simulink model "jointSpaceTrajController_reachPos"  (Simulink 8.0)
settings: Solver=FixedStepDiscrete  StartTime=0.0  StopTime=inf  FixedStep=Ts  RelTol=1e-3
undefined symbols (not defined in the file or in its folder): dqErr, qErr, qInit, qjDes, refMask, ROBOT_DOF
libraries: WBCLibrary x5
settings Model: Creator=nunoguedelha  LastModifiedBy=nunoguedelha

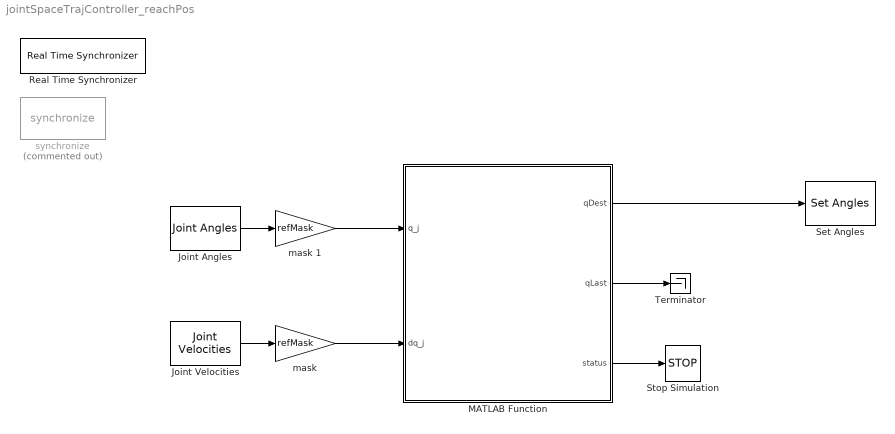
== system jointSpaceTrajController_reachPos ==
  Joint Angles : WBCLibrary/wholeBodyStates/Joint Angles  robotName=robotName  localName=localName
  Joint Velocities : WBCLibrary/wholeBodyStates/Joint Velocities  robotName=robotName  localName=localName
  MATLAB Function : MATLAB Function  TreatAsAtomicUnit=on
  Real Time Synchronizer : WBCLibrary/Utilities/Real Time Synchronizer  Priority=-10  threadPeriod=Ts
  Set Angles : WBCLibrary/wholeBodyActuators/Set Angles  val=5  robotName=robotName  localName=localName
  Stop Simulation : Stop
  Terminator : Terminator
  mask : Gain  Gain=refMask
  mask 1 : Gain  Gain=refMask
  synchronize : WBCLibrary/Utilities/synchronize  Commented=on  rate=0.010  scaleFactor=1
  wires:
  Joint Angles/1 -> mask 1/1
  Joint Velocities/1 -> mask/1
  mask 1/1 -> MATLAB Function/1(q_j)
  mask/1 -> MATLAB Function/2(dq_j)
  MATLAB Function/1(qDest) -> Set Angles/1
  MATLAB Function/2(qLast) -> Terminator/1
  MATLAB Function/3(status) -> Stop Simulation/1

== matlab function MATLAB Function ==
  data: qDest output double; qLast output double; qjDes parameter double; q_j input double; dq_j input double; qErr parameter double; dqErr parameter double; ROBOT_DOF parameter double; qInit parameter double; status output double; refMask parameter double
function [qDest, qLast, status] = checkStopCond(qjDes, q_j, dq_j, qErr, dqErr, ROBOT_DOF, qInit, refMask)
%#codegen

% Target position
qDest = qjDes.*refMask + qInit.*(ones(ROBOT_DOF,1)-refMask);

% Check if we reached the desired position:
% We shall stop as soon as |qDes-q_j| < qErr AND |dqDes-dq_j| < dqErr,
% qErr and dqErr being the approximative position and speed accuracy.
if norm((qjDes-q_j),Inf)<=qErr && norm(dq_j,Inf)<=dqErr
    status = 1;
else
    status = 0;
end

qLast = q_j;

end
